simulink model "verification"  (R2016b)
settings: Solver=FixedStepAuto  StartTime=0.0  StopTime=20  FixedStep=0.00001  RelTol=1e-3
settings Model: Creator=Niirn  LastModifiedBy=Niirn

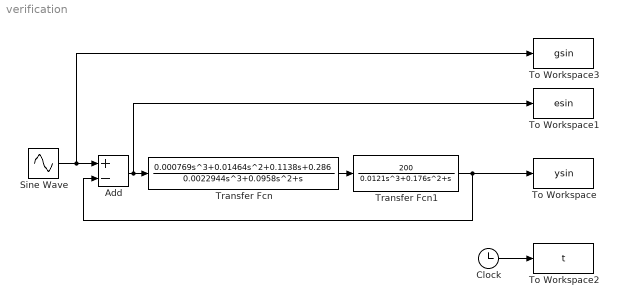
== system verification ==
  Add : Sum  Inputs=+-
  Clock : Clock
  Sine Wave : Sin  Amplitude=3.2  Frequency=0.5  SampleTime=0
  To Workspace : ToWorkspace  VariableName=ysin  SampleTime=-1
  To Workspace1 : ToWorkspace  VariableName=esin  SampleTime=-1
  To Workspace2 : ToWorkspace  VariableName=t  SampleTime=-1
  To Workspace3 : ToWorkspace  VariableName=gsin  SampleTime=-1
  Transfer Fcn : TransferFcn  Numerator=[0.000769 0.01464 0.1138 0.286]  Denominator=[0.0022944 0.0958 1 0]
  Transfer Fcn1 : TransferFcn  Numerator=[200]  Denominator=[0.0121 0.176 1 0]
  wires:
  Add/1 -> To Workspace1/1, Transfer Fcn/1
  Transfer Fcn/1 -> Transfer Fcn1/1
  Clock/1 -> To Workspace2/1
  Transfer Fcn1/1 -> To Workspace/1, Add/2
  Sine Wave/1 -> To Workspace3/1, Add/1
